simulink model "lab10simc"  (R2020a)
settings: Solver=VariableStepAuto  StartTime=0.0  StopTime=100  RelTol=1e-3
settings Model: Creator=ariana  LastModifiedBy=ariana

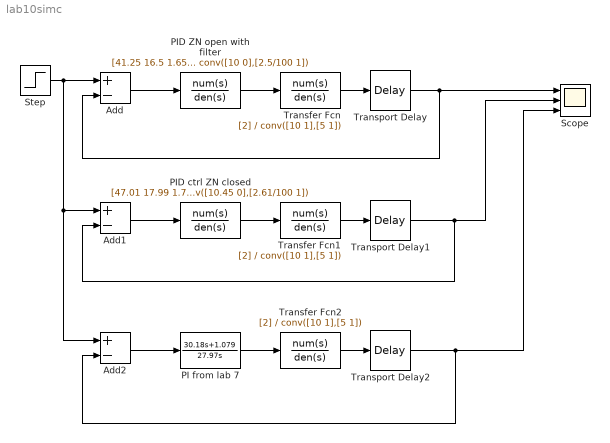
== system lab10simc ==
  Add : Sum  Inputs=+-
  Add1 : Sum  Inputs=+-
  Add2 : Sum  Inputs=+-
  PI from lab 7 : TransferFcn  Numerator=[30.18 1.079]  Denominator=[27.97 0]
  PID ZN open with filter : TransferFcn  Numerator=[41.25 16.5 1.65]  Denominator=conv([10 0],[2.5/100 1])
  PID ctrl ZN closed : TransferFcn  Numerator=[47.01 17.99 1.722]  Denominator=conv([10.45 0],[2.61/100 1])
  Scope : Scope  NumInputPorts=3
  Step : Step  Time=0  SampleTime=0
  Transfer Fcn : TransferFcn  Numerator=[2]  Denominator=conv([10 1],[5 1])
  Transfer Fcn1 : TransferFcn  Numerator=[2]  Denominator=conv([10 1],[5 1])
  Transfer Fcn2 : TransferFcn  Numerator=[2]  Denominator=conv([10 1],[5 1])
  Transport Delay : TransportDelay  DelayTime=3
  Transport Delay1 : TransportDelay  DelayTime=3
  Transport Delay2 : TransportDelay  DelayTime=3
  wires:
  Add/1 -> PID ZN open with filter/1
  PID ZN open with filter/1 -> Transfer Fcn/1
  Add1/1 -> PID ctrl ZN closed/1
  PID ctrl ZN closed/1 -> Transfer Fcn1/1
  Transfer Fcn1/1 -> Transport Delay1/1
  Transfer Fcn2/1 -> Transport Delay2/1
  PI from lab 7/1 -> Transfer Fcn2/1
  Add2/1 -> PI from lab 7/1
  Transfer Fcn/1 -> Transport Delay/1
  Step/1 -> Add2/1, Add1/1, Add/1
  Transport Delay/1 -> Add/2, Scope/1
  Transport Delay1/1 -> Add1/2, Scope/2
  Transport Delay2/1 -> Add2/2, Scope/3
